simulink model "SecRwLtStCalib"  (R2024b)
settings: Solver=FixedStepDiscrete  StartTime=0.0  StopTime=10.0  FixedStep=0.01  RelTol=1e-3
model workspace (MAT data in the model file):
  KeSMSwAcsMd6SecRwLtStBkReclnUpwdDnwdPos1Max_Val : Simulink.Parameter (value not decoded)
  KeSMSwAcsMd6SecRwLtStBkReclnUpwdDnwdPos1Min_Val : Simulink.Parameter (value not decoded)
  KeSMSwAcsMd6SecRwLtStBkReclnUpwdDnwdPos1_Val : Simulink.Parameter (value not decoded)
  KeSMSwAcsMd6SecRwLtStBkReclnUpwdDnwdPosMax_Val : Simulink.Parameter (value not decoded)
  KeSMSwAcsMd6SecRwLtStBkReclnUpwdDnwdPosMin_Val : Simulink.Parameter (value not decoded)
  KeSMSwAcsMd6SecRwLtStBkReclnUpwdDnwdPos_Val : Simulink.Parameter (value not decoded)
symbols that are objects in the model workspace (value not decoded): KeSMSwAcsMd6SecRwLtStBkReclnUpwdDnwdPos1_Val, KeSMSwAcsMd6SecRwLtStBkReclnUpwdDnwdPos1Max_Val, KeSMSwAcsMd6SecRwLtStBkReclnUpwdDnwdPos1Min_Val, KeSMSwAcsMd6SecRwLtStBkReclnUpwdDnwdPos_Val, KeSMSwAcsMd6SecRwLtStBkReclnUpwdDnwdPosMax_Val, KeSMSwAcsMd6SecRwLtStBkReclnUpwdDnwdPosMin_Val
undefined symbols (not defined in the file or in its folder): KeSMSw4SAcsMd21SecRwLtStBkReclnUpwdDnwdPos_Val, KeSMSw4SAcsMd21SecRwLtStBkReclnUpwdDnwdPosMax_Val, KeSMSw4SAcsMd21SecRwLtStBkReclnUpwdDnwdPosMin_Val, KeSMSw4SAcsMd21SecRwLtStFrwdBkwdPos_Val, KeSMSw4SAcsMd21SecRwLtStFrwdBkwdPosMax_Val, KeSMSw4SAcsMd21SecRwLtStFrwdBkwdPosMin_Val, KeSMSw4SAcsMd21SecRwLtStHdrstFrwdBkwdPos_Val, KeSMSw4SAcsMd21SecRwLtStHdrstFrwdBkwdPosMax_Val, KeSMSw4SAcsMd21SecRwLtStHdrstFrwdBkwdPosMin_Val, KeSMSw4SAcsMd21SecRwLtStHdrstUpwdDnwdPos_Val, KeSMSw4SAcsMd21SecRwLtStHdrstUpwdDnwdPosMax_Val, KeSMSw4SAcsMd21SecRwLtStHdrstUpwdDnwdPosMin_Val, KeSMSw4SAcsMd22SecRwLtStBkReclnUpwdDnwdPos1_Val, KeSMSw4SAcsMd22SecRwLtStBkReclnUpwdDnwdPos2_Val, KeSMSw4SAcsMd22SecRwLtStBkReclnUpwdDnwdPos2Max_Val, KeSMSw4SAcsMd22SecRwLtStBkReclnUpwdDnwdPos2Min_Val, KeSMSw4SAcsMd22SecRwLtStBkReclnUpwdDnwdPosMax_Val, KeSMSw4SAcsMd22SecRwLtStBkReclnUpwdDnwdPosMin_Val, KeSMSw4SAcsMd22SecRwLtStFrwdBkwdPos_Val, KeSMSw4SAcsMd22SecRwLtStFrwdBkwdPosMax_Val, KeSMSw4SAcsMd22SecRwLtStFrwdBkwdPosMin_Val, KeSMSw4SAcsMd22SecRwLtStFtrstUpwdDnwdPos_Val, KeSMSw4SAcsMd22SecRwLtStFtrstUpwdDnwdPosMax_Val, KeSMSw4SAcsMd22SecRwLtStFtrstUpwdDnwdPosMin_Val, KeSMSw4SAcsMd22SecRwLtStHdrstFrwdBkwdPos_Val, KeSMSw4SAcsMd22SecRwLtStHdrstFrwdBkwdPosMax_Val, KeSMSw4SAcsMd22SecRwLtStHdrstFrwdBkwdPosMin_Val, KeSMSw4SAcsMd22SecRwLtStHdrstUpwdDnwdPos_Val, KeSMSw4SAcsMd22SecRwLtStHdrstUpwdDnwdPosMax_Val, KeSMSw4SAcsMd22SecRwLtStHdrstUpwdDnwdPosMin_Val, KeSMSw4SAcsMd22SecRwLtStLegrstOtwdInwdPos_Val, KeSMSw4SAcsMd22SecRwLtStLegrstOtwdInwdPosMax_Val, KeSMSw4SAcsMd22SecRwLtStLegrstOtwdInwdPosMin_Val, KeSMSw4SAcsMd22SecRwLtStLegrstUpwdDnwdPos_Val, KeSMSw4SAcsMd22SecRwLtStLegrstUpwdDnwdPosMax_Val, KeSMSw4SAcsMd22SecRwLtStLegrstUpwdDnwdPosMin_Val, KeSMSw4SAcsMd25SecRwLtStBkReclnUpwdDnwdPos_Val, KeSMSw4SAcsMd25SecRwLtStBkReclnUpwdDnwdPosMax_Val, KeSMSw4SAcsMd25SecRwLtStBkReclnUpwdDnwdPosMin_Val, KeSMSw4SAcsMd25SecRwLtStFrwdBkwdPos_Val, KeSMSw4SAcsMd25SecRwLtStFrwdBkwdPosMax_Val, KeSMSw4SAcsMd25SecRwLtStFrwdBkwdPosMin_Val, KeSMSw4SAcsMd25SecRwLtStHdrstFrwdBkwdPos_Val, KeSMSw4SAcsMd25SecRwLtStHdrstFrwdBkwdPosMax_Val, KeSMSw4SAcsMd25SecRwLtStHdrstFrwdBkwdPosMin_Val, KeSMSw4SAcsMd25SecRwLtStHdrstUpwdDnwdPos_Val, KeSMSw4SAcsMd25SecRwLtStHdrstUpwdDnwdPosMax_Val, KeSMSw4SAcsMd25SecRwLtStHdrstUpwdDnwdPosMin_Val, KeSMSw4SAcsMd26SecRwLtStBkReclnUpwdDnwdPos_Val, KeSMSw4SAcsMd26SecRwLtStBkReclnUpwdDnwdPosMax_Val, KeSMSw4SAcsMd26SecRwLtStBkReclnUpwdDnwdPosMin_Val, KeSMSw4SAcsMd26SecRwLtStFrwdBkwdPos_Val, KeSMSw4SAcsMd26SecRwLtStFrwdBkwdPosMax_Val, KeSMSw4SAcsMd26SecRwLtStFrwdBkwdPosMin_Val, KeSMSw4SAcsMd26SecRwLtStFtrstUpwdDnwdPos_Val, KeSMSw4SAcsMd26SecRwLtStFtrstUpwdDnwdPosMax_Val, KeSMSw4SAcsMd26SecRwLtStFtrstUpwdDnwdPosMin_Val, KeSMSw4SAcsMd26SecRwLtStHdrstFrwdBkwdPos_Val, KeSMSw4SAcsMd26SecRwLtStHdrstFrwdBkwdPosMax_Val, KeSMSw4SAcsMd26SecRwLtStHdrstFrwdBkwdPosMin_Val ... (+496)
libraries: TrgtPosSelcLib x61, StIsPosChkLib x1, simulink x1
(part 2 of 8)

== system SecRwLtStCalib/SecRwLtStArmScrnTrgtPosSelc_1_Cal_sys ==
  StNumFlg_Is4s_read : Inport
  StNumFlg_Is6s_read : Inport  Port=2
  StNumFlg_Is6s7s_read : Inport  Port=3
  StNumFlg_Is7s_read : Inport  Port=4
  function : TriggerPort  TriggerType=function-call  IsSimulinkFunction=on  FunctionName=SecRwLtStArmScrnTrgtPosSelc_1_Cal  VariantControl=(inherit)
  Ground_1 : Ground
  Ground_2 : Ground
  Terminator_{1..4} (4 alike) : Terminator
  EZER2LArmScrnTrgtPosCalib_TrgtPosArray_write : Outport  VectorParamsAs1DForOutWhenUnconnected=off
      settings: EnsureOutportIsVirtual=on
  EZQR2LArmScrnTrgtPosCalib_TrgtPosArray_write : Outport  Port=2  VectorParamsAs1DForOutWhenUnconnected=off
      settings: EnsureOutportIsVirtual=on
  wires:
  StNumFlg_Is4s_read/1 -> Terminator_1/1
  StNumFlg_Is6s_read/1 -> Terminator_2/1
  StNumFlg_Is6s7s_read/1 -> Terminator_3/1
  StNumFlg_Is7s_read/1 -> Terminator_4/1
  Ground_1/1 -> EZER2LArmScrnTrgtPosCalib_TrgtPosArray_write/1
  Ground_2/1 -> EZQR2LArmScrnTrgtPosCalib_TrgtPosArray_write/1

== system SecRwLtStCalib/SecRwLtStBkReclnTrgtPosSelc_1_Cal_sys ==
  IfVeSMSbSecRwLtStCshnFrntUpwdDnwdMovConfig_Val_read : Inport
  IfVeSMSuThdRwLtStCshnFldUpwdDnwdPos_Val_read : Inport  Port=2
  modestate32_Val_read : Inport  Port=3
  R2LBkReclinFirstStepPassFlg_Val_read : Inport  Port=4
  R2LMdSeatOccupied_Val_read : Inport  Port=5
  StNumFlg_Is4s_read : Inport  Port=6
  StNumFlg_Is6s_read : Inport  Port=7
  StNumFlg_Is6s7s_read : Inport  Port=8
  StNumFlg_Is7s_read : Inport  Port=9
  ThdRwLtStCshnFldStgDone_Val_read : Inport  Port=10
  Md27Target1_Val_read : Inport  Port=11
  Md27Target2_Val_read : Inport  Port=12
  function : TriggerPort  TriggerType=function-call  IsSimulinkFunction=on  FunctionName=SecRwLtStBkReclnTrgtPosSelc_1_Cal  VariantControl=(inherit)
  Subsystem1 : Subsystem
  EZER2LBkReclnUpwdDnwdTrgtPosCalib_TrgtPosArray_write : Outport  VectorParamsAs1DForOutWhenUnconnected=off
  EZER2LBkReclnUpwdDnwdTrgtPosCalib1_TrgtPosArray_write : Outport  Port=2  VectorParamsAs1DForOutWhenUnconnected=off
  EZQR2LBkReclnUpwdDnwdTrgtPosCalib_TrgtPosArray_write : Outport  Port=3  VectorParamsAs1DForOutWhenUnconnected=off
  KeSMSw4SAcsMd21BkReclnUpwdDnwdTrgtPosCalib_TrgtPosArray_write : Outport  Port=4  VectorParamsAs1DForOutWhenUnconnected=off
  KeSMSw4SAcsMd22BkReclnUpwdDnwdTrgtPosCalib_TrgtPosArray_write : Outport  Port=5  VectorParamsAs1DForOutWhenUnconnected=off
  KeSMSw4SAcsMd25BkReclnUpwdDnwdTrgtPosCalib_TrgtPosArray_write : Outport  Port=6  VectorParamsAs1DForOutWhenUnconnected=off
  KeSMSw4SAcsMd26BkReclnUpwdDnwdTrgtPosCalib_TrgtPosArray_write : Outport  Port=7  VectorParamsAs1DForOutWhenUnconnected=off
  KeSMSwMd32R2LBkReclnUpwdDnwdTrgtPosCalib_TrgtPosArray_write : Outport  Port=8  VectorParamsAs1DForOutWhenUnconnected=off
  LyLR2LBkReclnUpwdDnwdTrgtPosCalib_TrgtPosArray_write : Outport  Port=9  VectorParamsAs1DForOutWhenUnconnected=off
  Md56R2LBkReclnUpwdDnwdTrgtPosCalib_TrgtPosArray_write : Outport  Port=10  VectorParamsAs1DForOutWhenUnconnected=off
  Md56R2LBkReclnUpwdDnwdTrgtPosCalib1_TrgtPosArray_write : Outport  Port=11  VectorParamsAs1DForOutWhenUnconnected=off
  Md8R2LBkReclnUpwdDnwdTrgtPosCalib_TrgtPosArray_write : Outport  Port=12  VectorParamsAs1DForOutWhenUnconnected=off
  RecvLR2LBkReclnUpwdDnwdTrgtPosCalib_TrgtPosArray_write : Outport  Port=13  VectorParamsAs1DForOutWhenUnconnected=off
  SecRwLtStBkReclnEnTrigBitMask_Val_write : Outport  Port=14  VectorParamsAs1DForOutWhenUnconnected=off
  VIPLExitR2LBkReclnUpwdDnwdTrgtPosCalib_TrgtPosArray_write : Outport  Port=15  VectorParamsAs1DForOutWhenUnconnected=off
  VIPLR2LBkReclnUpwdDnwdTrgtPosCalib_TrgtPosArray_write : Outport  Port=16  VectorParamsAs1DForOutWhenUnconnected=off
  Md27SecRwLtStBkReclnTrgtPosCalib_TrgtPosArray_write : Outport  Port=17  VectorParamsAs1DForOutWhenUnconnected=off
      settings: EnsureOutportIsVirtual=on
  wires:
  Subsystem1/16(SecRwLtStBkReclnEnTrigBitMask_Val_write) -> SecRwLtStBkReclnEnTrigBitMask_Val_write/1
  Subsystem1/1(EZER2LBkReclnUpwdDnwdTrgtPosCalib_TrgtPosArray_write) -> EZER2LBkReclnUpwdDnwdTrgtPosCalib_TrgtPosArray_write/1
  Subsystem1/2(EZQR2LBkReclnUpwdDnwdTrgtPosCalib_TrgtPosArray_write) -> EZQR2LBkReclnUpwdDnwdTrgtPosCalib_TrgtPosArray_write/1
  Subsystem1/3(KeSMSw4SAcsMd21BkReclnUpwdDnwdTrgtPosCalib_TrgtPosArray_write) -> KeSMSw4SAcsMd21BkReclnUpwdDnwdTrgtPosCalib_TrgtPosArray_write/1
  Subsystem1/4(KeSMSw4SAcsMd22BkReclnUpwdDnwdTrgtPosCalib_TrgtPosArray_write) -> KeSMSw4SAcsMd22BkReclnUpwdDnwdTrgtPosCalib_TrgtPosArray_write/1
  Subsystem1/5(KeSMSw4SAcsMd25BkReclnUpwdDnwdTrgtPosCalib_TrgtPosArray_write) -> KeSMSw4SAcsMd25BkReclnUpwdDnwdTrgtPosCalib_TrgtPosArray_write/1
  Subsystem1/6(KeSMSw4SAcsMd26BkReclnUpwdDnwdTrgtPosCalib_TrgtPosArray_write) -> KeSMSw4SAcsMd26BkReclnUpwdDnwdTrgtPosCalib_TrgtPosArray_write/1
  Subsystem1/7(LyLR2LBkReclnUpwdDnwdTrgtPosCalib_TrgtPosArray_write) -> LyLR2LBkReclnUpwdDnwdTrgtPosCalib_TrgtPosArray_write/1
  Subsystem1/8(RecvLR2LBkReclnUpwdDnwdTrgtPosCalib_TrgtPosArray_write) -> RecvLR2LBkReclnUpwdDnwdTrgtPosCalib_TrgtPosArray_write/1
  Subsystem1/9(VIPLR2LBkReclnUpwdDnwdTrgtPosCalib_TrgtPosArray_write) -> VIPLR2LBkReclnUpwdDnwdTrgtPosCalib_TrgtPosArray_write/1
  Subsystem1/10(EZER2LBkReclnUpwdDnwdTrgtPosCalib1_TrgtPosArray_write) -> EZER2LBkReclnUpwdDnwdTrgtPosCalib1_TrgtPosArray_write/1
  Subsystem1/11(VIPLExitR2LBkReclnUpwdDnwdTrgtPosCalib_TrgtPosArray_write) -> VIPLExitR2LBkReclnUpwdDnwdTrgtPosCalib_TrgtPosArray_write/1
  Subsystem1/12(KeSMSwMd32R2LBkReclnUpwdDnwdTrgtPosCalib_TrgtPosArray_write) -> KeSMSwMd32R2LBkReclnUpwdDnwdTrgtPosCalib_TrgtPosArray_write/1
  Subsystem1/13(Md8R2LBkReclnUpwdDnwdTrgtPosCalib_TrgtPosArray_write) -> Md8R2LBkReclnUpwdDnwdTrgtPosCalib_TrgtPosArray_write/1
  Subsystem1/15(Md56R2LBkReclnUpwdDnwdTrgtPosCalib1_TrgtPosArray_write) -> Md56R2LBkReclnUpwdDnwdTrgtPosCalib1_TrgtPosArray_write/1
  Subsystem1/14(Md56R2LBkReclnUpwdDnwdTrgtPosCalib_TrgtPosArray_write) -> Md56R2LBkReclnUpwdDnwdTrgtPosCalib_TrgtPosArray_write/1
  IfVeSMSbSecRwLtStCshnFrntUpwdDnwdMovConfig_Val_read/1 -> Subsystem1/8(IfVeSMSbSecRwLtStCshnFrntUpwdDnwdMovConfig_Val_read)
  IfVeSMSuThdRwLtStCshnFldUpwdDnwdPos_Val_read/1 -> Subsystem1/10(IfVeSMSuThdRwLtStCshnFldUpwdDnwdPos_Val_read)
  ThdRwLtStCshnFldStgDone_Val_read/1 -> Subsystem1/9(ThdRwLtStCshnFldStgDone_Val_read)
  R2LBkReclinFirstStepPassFlg_Val_read/1 -> Subsystem1/7(R2LBkReclinFirstStepPassFlg_Val_read)
  modestate32_Val_read/1 -> Subsystem1/6(modestate32_Val_read)
  R2LMdSeatOccupied_Val_read/1 -> Subsystem1/5(R2LMdSeatOccupied_Val_read)
  StNumFlg_Is4s_read/1 -> Subsystem1/1(StNumFlg_Is4s_read)
  StNumFlg_Is7s_read/1 -> Subsystem1/4(StNumFlg_Is7s_read)
  StNumFlg_Is6s7s_read/1 -> Subsystem1/3(StNumFlg_Is6s7s_read)
  StNumFlg_Is6s_read/1 -> Subsystem1/2(StNumFlg_Is6s_read)
  Md27Target1_Val_read/1 -> Subsystem1/11(Md27Target1_Val_read)
  Md27Target2_Val_read/1 -> Subsystem1/12(Md27Target2_Val_read)
  Subsystem1/17(Md27SecRwLtStBkReclnTrgtPosCalib_TrgtPosArray_write) -> Md27SecRwLtStBkReclnTrgtPosCalib_TrgtPosArray_write/1

== system SecRwLtStCalib/SecRwLtStCalib_Init ==
  Event Listener : EventListener  EventName=reset

== system SecRwLtStCalib/SecRwLtStFtrstTrgtPosSelc_1_Cal_sys ==
  StNumFlg_Is4s_read : Inport
  StNumFlg_Is6s_read : Inport  Port=2
  StNumFlg_Is6s7s_read : Inport  Port=3
  StNumFlg_Is7s_read : Inport  Port=4
  function : TriggerPort  TriggerType=function-call  IsSimulinkFunction=on  FunctionName=SecRwLtStFtrstTrgtPosSelc_1_Cal  VariantControl=(inherit)
  Ground_{1..7} (7 alike) : Ground
  Terminator_{1..4} (4 alike) : Terminator
  KeSMSw4SAcsMd22FtrstTrgtPosCalib_TrgtPosArray_write : Outport  VectorParamsAs1DForOutWhenUnconnected=off
      settings: EnsureOutportIsVirtual=on
  KeSMSw4SAcsMd26FtrstTrgtPosCalib_TrgtPosArray_write : Outport  Port=2  VectorParamsAs1DForOutWhenUnconnected=off
      settings: EnsureOutportIsVirtual=on
  LgrstCloseLR2LFtrstTrgtPosCalib_TrgtPosArray_write : Outport  Port=3  VectorParamsAs1DForOutWhenUnconnected=off
      settings: EnsureOutportIsVirtual=on
  LgrstOpenLR2LFtrstTrgtPosCalib_TrgtPosArray_write : Outport  Port=4  VectorParamsAs1DForOutWhenUnconnected=off
      settings: EnsureOutportIsVirtual=on
  LyLR2LFtrstTrgtPosCalib_TrgtPosArray_write : Outport  Port=5  VectorParamsAs1DForOutWhenUnconnected=off
      settings: EnsureOutportIsVirtual=on
  RecvLR2LFtrstTrgtPosCalib_TrgtPosArray_write : Outport  Port=6  VectorParamsAs1DForOutWhenUnconnected=off
      settings: EnsureOutportIsVirtual=on
  VIPLR2LFtrstTrgtPosCalib_TrgtPosArray_write : Outport  Port=7  VectorParamsAs1DForOutWhenUnconnected=off
      settings: EnsureOutportIsVirtual=on
  wires:
  StNumFlg_Is4s_read/1 -> Terminator_1/1
  StNumFlg_Is6s_read/1 -> Terminator_2/1
  StNumFlg_Is6s7s_read/1 -> Terminator_3/1
  StNumFlg_Is7s_read/1 -> Terminator_4/1
  Ground_1/1 -> KeSMSw4SAcsMd22FtrstTrgtPosCalib_TrgtPosArray_write/1
  Ground_2/1 -> KeSMSw4SAcsMd26FtrstTrgtPosCalib_TrgtPosArray_write/1
  Ground_3/1 -> LgrstCloseLR2LFtrstTrgtPosCalib_TrgtPosArray_write/1
  Ground_4/1 -> LgrstOpenLR2LFtrstTrgtPosCalib_TrgtPosArray_write/1
  Ground_5/1 -> LyLR2LFtrstTrgtPosCalib_TrgtPosArray_write/1
  Ground_6/1 -> RecvLR2LFtrstTrgtPosCalib_TrgtPosArray_write/1
  Ground_7/1 -> VIPLR2LFtrstTrgtPosCalib_TrgtPosArray_write/1

== system SecRwLtStCalib/SecRwLtStFwdBkwdTrgtPosSelc_1_Cal_sys ==
  note: Added blocks
  note: Added blocks
  note: Added blocks
  IfVeSMSbSecRwLtStCshnFrntUpwdDnwdMovConfig_Val_read : Inport
  IfVeSMSuSecRwRtStFrwdBkwdPos_Val_read : Inport  Port=2
  IfVeSMSuSecRwRtStFrwdBkwdPosV_Val_read : Inport  Port=3
  StNumFlg_Is4s_read : Inport  Port=4
  StNumFlg_Is6s_read : Inport  Port=5
  StNumFlg_Is6s7s_read : Inport  Port=6
  StNumFlg_Is7s_read : Inport  Port=7
  function : TriggerPort  TriggerType=function-call  IsSimulinkFunction=on  FunctionName=SecRwLtStFwdBkwdTrgtPosSelc_1_Cal  VariantControl=(inherit)
  PA_KeSMSwAcsMd6SecRwLtStBkReclnUpwdDnwdPos1Max_Val : Constant  Value=KeSMSwAcsMd6SecRwLtStBkReclnUpwdDnwdPos1Max_Val
  PA_KeSMSwAcsMd6SecRwLtStBkReclnUpwdDnwdPos1Min_Val : Constant  Value=KeSMSwAcsMd6SecRwLtStBkReclnUpwdDnwdPos1Min_Val
  PA_KeSMSwAcsMd6SecRwLtStBkReclnUpwdDnwdPos1_Val : Constant  Value=KeSMSwAcsMd6SecRwLtStBkReclnUpwdDnwdPos1_Val
  PA_KeSMSwAcsMd6SecRwLtStBkReclnUpwdDnwdPosMax_Val : Constant  Value=KeSMSwAcsMd6SecRwLtStBkReclnUpwdDnwdPosMax_Val
  PA_KeSMSwAcsMd6SecRwLtStBkReclnUpwdDnwdPosMin_Val : Constant  Value=KeSMSwAcsMd6SecRwLtStBkReclnUpwdDnwdPosMin_Val
  Subsystem2 : Subsystem
  Terminator_{495..499} (5 alike) : Terminator
  EZER2LFwdBkwdTrgtPosCalib_TrgtPosArray_write : Outport  VectorParamsAs1DForOutWhenUnconnected=off
  EZQR2LFwdBkwdTrgtPosCalib_TrgtPosArray_write : Outport  Port=2  VectorParamsAs1DForOutWhenUnconnected=off
  FamlyLR2LFwdBkwdTrgtPosCalib_TrgtPosArray_write : Outport  Port=3  VectorParamsAs1DForOutWhenUnconnected=off
  FamlyRR2LFwdBkwdTrgtPosCalib_TrgtPosArray_write : Outport  Port=4  VectorParamsAs1DForOutWhenUnconnected=off
  INTMLR2LFwdBkwdTrgtPosCalib_TrgtPosArray_write : Outport  Port=5  VectorParamsAs1DForOutWhenUnconnected=off
  KeSMSw4SAcsMd21FwdBkwdTrgtPosCalib_TrgtPosArray_write : Outport  Port=6  VectorParamsAs1DForOutWhenUnconnected=off
  KeSMSw4SAcsMd22FwdBkwdTrgtPosCalib_TrgtPosArray_write : Outport  Port=7  VectorParamsAs1DForOutWhenUnconnected=off
  KeSMSw4SAcsMd25FwdBkwdTrgtPosCalib_TrgtPosArray_write : Outport  Port=8  VectorParamsAs1DForOutWhenUnconnected=off
  KeSMSw4SAcsMd26FwdBkwdTrgtPosCalib_TrgtPosArray_write : Outport  Port=9  VectorParamsAs1DForOutWhenUnconnected=off
  KeSMSw4sLegrstOpenLMdFwdBkwdTrgtPosCalib_TrgtPosArray_write : Outport  Port=10  VectorParamsAs1DForOutWhenUnconnected=off
  KeSMSw4SLyingLMDFwdBkwdTrgtPosCalib_TrgtPosArray_write : Outport  Port=11  VectorParamsAs1DForOutWhenUnconnected=off
  KeSMSw4SVIPLMDFwdBkwdTrgtPosCalib_TrgtPosArray_write : Outport  Port=12  VectorParamsAs1DForOutWhenUnconnected=off
  Md56R2LFwdBkwdTrgtPosCalib_TrgtPosArray_write : Outport  Port=13  VectorParamsAs1DForOutWhenUnconnected=off
  Md8R2LFwdBkwdTrgtPosCalib_TrgtPosArray_write : Outport  Port=14  VectorParamsAs1DForOutWhenUnconnected=off
  SecRwLtStFwdBkwdEnTrigBitMask_Val_write : Outport  Port=15  VectorParamsAs1DForOutWhenUnconnected=off
  VIPLExitR2LFwdBkwdTrgtPosCalib_TrgtPosArray_write : Outport  Port=16  VectorParamsAs1DForOutWhenUnconnected=off
  VIPLR2LFwdBkwdTrgtPosCalib_TrgtPosArray_write : Outport  Port=17  VectorParamsAs1DForOutWhenUnconnected=off
  wires:
  Subsystem2/17(SecRwLtStFwdBkwdEnTrigBitMask_Val_write) -> SecRwLtStFwdBkwdEnTrigBitMask_Val_write/1
  Subsystem2/1(EZER2LFwdBkwdTrgtPosCalib_TrgtPosArray_write) -> EZER2LFwdBkwdTrgtPosCalib_TrgtPosArray_write/1
  Subsystem2/2(EZQR2LFwdBkwdTrgtPosCalib_TrgtPosArray_write) -> EZQR2LFwdBkwdTrgtPosCalib_TrgtPosArray_write/1
  Subsystem2/3(FamlyLR2LFwdBkwdTrgtPosCalib_TrgtPosArray_write) -> FamlyLR2LFwdBkwdTrgtPosCalib_TrgtPosArray_write/1
  Subsystem2/4(FamlyRR2LFwdBkwdTrgtPosCalib_TrgtPosArray_write) -> FamlyRR2LFwdBkwdTrgtPosCalib_TrgtPosArray_write/1
  Subsystem2/5(INTMLR2LFwdBkwdTrgtPosCalib_TrgtPosArray_write) -> INTMLR2LFwdBkwdTrgtPosCalib_TrgtPosArray_write/1
  Subsystem2/6(KeSMSw4SAcsMd21FwdBkwdTrgtPosCalib_TrgtPosArray_write) -> KeSMSw4SAcsMd21FwdBkwdTrgtPosCalib_TrgtPosArray_write/1
  Subsystem2/7(KeSMSw4SAcsMd22FwdBkwdTrgtPosCalib_TrgtPosArray_write) -> KeSMSw4SAcsMd22FwdBkwdTrgtPosCalib_TrgtPosArray_write/1
  Subsystem2/8(KeSMSw4SAcsMd25FwdBkwdTrgtPosCalib_TrgtPosArray_write) -> KeSMSw4SAcsMd25FwdBkwdTrgtPosCalib_TrgtPosArray_write/1
  Subsystem2/9(KeSMSw4SAcsMd26FwdBkwdTrgtPosCalib_TrgtPosArray_write) -> KeSMSw4SAcsMd26FwdBkwdTrgtPosCalib_TrgtPosArray_write/1
  Subsystem2/10(VIPLR2LFwdBkwdTrgtPosCalib_TrgtPosArray_write) -> VIPLR2LFwdBkwdTrgtPosCalib_TrgtPosArray_write/1
  Subsystem2/11(KeSMSw4sLegrstOpenLMdFwdBkwdTrgtPosCalib_TrgtPosArray_write) -> KeSMSw4sLegrstOpenLMdFwdBkwdTrgtPosCalib_TrgtPosArray_write/1
  Subsystem2/12(KeSMSw4SLyingLMDFwdBkwdTrgtPosCalib_TrgtPosArray_write) -> KeSMSw4SLyingLMDFwdBkwdTrgtPosCalib_TrgtPosArray_write/1
  Subsystem2/16(Md56R2LFwdBkwdTrgtPosCalib_TrgtPosArray_write) -> Md56R2LFwdBkwdTrgtPosCalib_TrgtPosArray_write/1
  Subsystem2/15(Md8R2LFwdBkwdTrgtPosCalib_TrgtPosArray_write) -> Md8R2LFwdBkwdTrgtPosCalib_TrgtPosArray_write/1
  Subsystem2/14(VIPLExitR2LFwdBkwdTrgtPosCalib_TrgtPosArray_write) -> VIPLExitR2LFwdBkwdTrgtPosCalib_TrgtPosArray_write/1
  Subsystem2/13(KeSMSw4SVIPLMDFwdBkwdTrgtPosCalib_TrgtPosArray_write) -> KeSMSw4SVIPLMDFwdBkwdTrgtPosCalib_TrgtPosArray_write/1
  IfVeSMSuSecRwRtStFrwdBkwdPos_Val_read/1 -> Subsystem2/1(IfVeSMSuSecRwRtStFrwdBkwdPos_Val_read)
  IfVeSMSuSecRwRtStFrwdBkwdPosV_Val_read/1 -> Subsystem2/2(IfVeSMSuSecRwRtStFrwdBkwdPosV_Val_read)
  StNumFlg_Is4s_read/1 -> Subsystem2/3(StNumFlg_Is4s_read)
  StNumFlg_Is6s_read/1 -> Subsystem2/4(StNumFlg_Is6s_read)
  StNumFlg_Is6s7s_read/1 -> Subsystem2/5(StNumFlg_Is6s7s_read)
  StNumFlg_Is7s_read/1 -> Subsystem2/6(StNumFlg_Is7s_read)
  IfVeSMSbSecRwLtStCshnFrntUpwdDnwdMovConfig_Val_read/1 -> Subsystem2/7(IfVeSMSbSecRwLtStCshnFrntUpwdDnwdMovConfig_Val_read)

== system SecRwLtStCalib/SecRwLtStHdrstFwdBkwdTrgtPosSelc_1_Cal_sys ==
  IfVeSMSuHeightIndexLt_Val_read : Inport
  StNumFlg_Is4s_read : Inport  Port=2
  StNumFlg_Is6s_read : Inport  Port=3
  StNumFlg_Is6s7s_read : Inport  Port=4
  StNumFlg_Is7s_read : Inport  Port=5
  function : TriggerPort  TriggerType=function-call  IsSimulinkFunction=on  FunctionName=SecRwLtStHdrstFwdBkwdTrgtPosSelc_1_Cal  VariantControl=(inherit)
  Ground_{1..7} (7 alike) : Ground
  Terminator_{1..5} (5 alike) : Terminator
  KeSMSw4SAcsMd21HdrstFwdBkwdTrgtPosCalib_TrgtPosArray_write : Outport  VectorParamsAs1DForOutWhenUnconnected=off
      settings: EnsureOutportIsVirtual=on
  KeSMSw4SAcsMd22HdrstFwdBkwdTrgtPosCalib_TrgtPosArray_write : Outport  Port=2  VectorParamsAs1DForOutWhenUnconnected=off
      settings: EnsureOutportIsVirtual=on
  KeSMSw4SAcsMd25HdrstFwdBkwdTrgtPosCalib_TrgtPosArray_write : Outport  Port=3  VectorParamsAs1DForOutWhenUnconnected=off
      settings: EnsureOutportIsVirtual=on
  KeSMSw4SAcsMd26HdrstFwdBkwdTrgtPosCalib_TrgtPosArray_write : Outport  Port=4  VectorParamsAs1DForOutWhenUnconnected=off
      settings: EnsureOutportIsVirtual=on
  LyLR2LHdrstFwdBkwdTrgtPosCalib_TrgtPosArray_write : Outport  Port=5  VectorParamsAs1DForOutWhenUnconnected=off
      settings: EnsureOutportIsVirtual=on
  RecvLR2LHdrstFwdBkwdTrgtPosCalib_TrgtPosArray_write : Outport  Port=6  VectorParamsAs1DForOutWhenUnconnected=off
      settings: EnsureOutportIsVirtual=on
  VIPLR2LHdrstFwdBkwdTrgtPosCalib_TrgtPosArray_write : Outport  Port=7  VectorParamsAs1DForOutWhenUnconnected=off
      settings: EnsureOutportIsVirtual=on
  wires:
  IfVeSMSuHeightIndexLt_Val_read/1 -> Terminator_1/1
  StNumFlg_Is4s_read/1 -> Terminator_2/1
  StNumFlg_Is6s_read/1 -> Terminator_3/1
  StNumFlg_Is6s7s_read/1 -> Terminator_4/1
  StNumFlg_Is7s_read/1 -> Terminator_5/1
  Ground_1/1 -> KeSMSw4SAcsMd21HdrstFwdBkwdTrgtPosCalib_TrgtPosArray_write/1
  Ground_2/1 -> KeSMSw4SAcsMd22HdrstFwdBkwdTrgtPosCalib_TrgtPosArray_write/1
  Ground_3/1 -> KeSMSw4SAcsMd25HdrstFwdBkwdTrgtPosCalib_TrgtPosArray_write/1
  Ground_4/1 -> KeSMSw4SAcsMd26HdrstFwdBkwdTrgtPosCalib_TrgtPosArray_write/1
  Ground_5/1 -> LyLR2LHdrstFwdBkwdTrgtPosCalib_TrgtPosArray_write/1
  Ground_6/1 -> RecvLR2LHdrstFwdBkwdTrgtPosCalib_TrgtPosArray_write/1
  Ground_7/1 -> VIPLR2LHdrstFwdBkwdTrgtPosCalib_TrgtPosArray_write/1

== system SecRwLtStCalib/SecRwLtStHdrstUpwdDnwdTrgtPosSelc_1_Cal_sys ==
  IfVeSMSuHeightIndexLt_Val_read : Inport
  StNumFlg_Is4s_read : Inport  Port=2
  StNumFlg_Is6s_read : Inport  Port=3
  StNumFlg_Is6s7s_read : Inport  Port=4
  StNumFlg_Is7s_read : Inport  Port=5
  function : TriggerPort  TriggerType=function-call  IsSimulinkFunction=on  FunctionName=SecRwLtStHdrstUpwdDnwdTrgtPosSelc_1_Cal  VariantControl=(inherit)
  Ground_{1..7} (7 alike) : Ground
  Terminator_{1..5} (5 alike) : Terminator
  KeSMSw4SAcsMd21HdrstUpwdDnwdTrgtPosCalib_TrgtPosArray_write : Outport  VectorParamsAs1DForOutWhenUnconnected=off
      settings: EnsureOutportIsVirtual=on
  KeSMSw4SAcsMd22HdrstUpwdDnwdTrgtPosCalib_TrgtPosArray_write : Outport  Port=2  VectorParamsAs1DForOutWhenUnconnected=off
      settings: EnsureOutportIsVirtual=on
  KeSMSw4SAcsMd25HdrstUpwdDnwdTrgtPosCalib_TrgtPosArray_write : Outport  Port=3  VectorParamsAs1DForOutWhenUnconnected=off
      settings: EnsureOutportIsVirtual=on
  KeSMSw4SAcsMd26HdrstUpwdDnwdTrgtPosCalib_TrgtPosArray_write : Outport  Port=4  VectorParamsAs1DForOutWhenUnconnected=off
      settings: EnsureOutportIsVirtual=on
  LyLR2LHdrstUpwdDnwdTrgtPosCalib_TrgtPosArray_write : Outport  Port=5  VectorParamsAs1DForOutWhenUnconnected=off
      settings: EnsureOutportIsVirtual=on
  RecvLR2LHdrstUpwdDnwdTrgtPosCalib_TrgtPosArray_write : Outport  Port=6  VectorParamsAs1DForOutWhenUnconnected=off
      settings: EnsureOutportIsVirtual=on
  VIPLR2LHdrstUpwdDnwdTrgtPosCalib_TrgtPosArray_write : Outport  Port=7  VectorParamsAs1DForOutWhenUnconnected=off
      settings: EnsureOutportIsVirtual=on
  wires:
  IfVeSMSuHeightIndexLt_Val_read/1 -> Terminator_1/1
  StNumFlg_Is4s_read/1 -> Terminator_2/1
  StNumFlg_Is6s_read/1 -> Terminator_3/1
  StNumFlg_Is6s7s_read/1 -> Terminator_4/1
  StNumFlg_Is7s_read/1 -> Terminator_5/1
  Ground_1/1 -> KeSMSw4SAcsMd21HdrstUpwdDnwdTrgtPosCalib_TrgtPosArray_write/1
  Ground_2/1 -> KeSMSw4SAcsMd22HdrstUpwdDnwdTrgtPosCalib_TrgtPosArray_write/1
  Ground_3/1 -> KeSMSw4SAcsMd25HdrstUpwdDnwdTrgtPosCalib_TrgtPosArray_write/1
  Ground_4/1 -> KeSMSw4SAcsMd26HdrstUpwdDnwdTrgtPosCalib_TrgtPosArray_write/1
  Ground_5/1 -> LyLR2LHdrstUpwdDnwdTrgtPosCalib_TrgtPosArray_write/1
  Ground_6/1 -> RecvLR2LHdrstUpwdDnwdTrgtPosCalib_TrgtPosArray_write/1
  Ground_7/1 -> VIPLR2LHdrstUpwdDnwdTrgtPosCalib_TrgtPosArray_write/1

== system SecRwLtStCalib/SecRwLtStLgrstInwdOtwdTrgtPosSelc_1_Cal_sys ==
  IfVeSMSbSecRwLtStCshnFrntUpwdDnwdMovConfig_Val_read : Inport
  IfVeSMSuHeightIndexLt_Val_read : Inport  Port=2
  StNumFlg_Is4s_read : Inport  Port=3
  StNumFlg_Is6s_read : Inport  Port=4
  StNumFlg_Is6s7s_read : Inport  Port=5
  StNumFlg_Is7s_read : Inport  Port=6
  function : TriggerPort  TriggerType=function-call  IsSimulinkFunction=on  FunctionName=SecRwLtStLgrstInwdOtwdTrgtPosSelc_1_Cal  VariantControl=(inherit)
  Subsystem2 : Subsystem
  KeSMSw4SAcsMd22LgrstInwdOtwdTrgtPosCalib_TrgtPosArray_write : Outport  VectorParamsAs1DForOutWhenUnconnected=off
  KeSMSw4SAcsMd26LgrstInwdOtwdTrgtPosCalib_TrgtPosArray_write : Outport  Port=2  VectorParamsAs1DForOutWhenUnconnected=off
  KeSMSwEZEEntryLgrstInwdOtwdTrgtPosCalib_TrgtPosArray_write : Outport  Port=3  VectorParamsAs1DForOutWhenUnconnected=off
  LgrstCloseLR2LLgrstInwdOtwdTrgtPosCalib_TrgtPosArray_write : Outport  Port=4  VectorParamsAs1DForOutWhenUnconnected=off
  LgrstOpen4sLR2LLgrstInwdOtwdTrgtPosCalib_TrgtPosArray_write : Outport  Port=5  VectorParamsAs1DForOutWhenUnconnected=off
  LyLR2LLgrstInwdOtwdTrgtPosCalib_TrgtPosArray_write : Outport  Port=6  VectorParamsAs1DForOutWhenUnconnected=off
  Md56LgrstInwdOtwdTrgtPosCalib_TrgtPosArray_write : Outport  Port=7  VectorParamsAs1DForOutWhenUnconnected=off
  Md8R2LLgrstInwdOtwdTrgtPosCalib_TrgtPosArray_write : Outport  Port=8  VectorParamsAs1DForOutWhenUnconnected=off
  RecvLR2LLgrstInwdOtwdTrgtPosCalib_TrgtPosArray_write : Outport  Port=9  VectorParamsAs1DForOutWhenUnconnected=off
  SecRwLtStLgrstInwdOtwdEnTrigBitMask_Val_write : Outport  Port=10  VectorParamsAs1DForOutWhenUnconnected=off
  VIP4sLR2LLgrstInwdOtwdTrgtPosCalib_TrgtPosArray_write : Outport  Port=11  VectorParamsAs1DForOutWhenUnconnected=off
  VIPLExitR2LLgrstInwdOtwdTrgtPosCalib_TrgtPosArray_write : Outport  Port=12  VectorParamsAs1DForOutWhenUnconnected=off
  VIPLR2LLgrstInwdOtwdTrgtPosCalib_TrgtPosArray_write : Outport  Port=13  VectorParamsAs1DForOutWhenUnconnected=off
  wires:
  Subsystem2/13(SecRwLtStLgrstInwdOtwdEnTrigBitMask_Val_write) -> SecRwLtStLgrstInwdOtwdEnTrigBitMask_Val_write/1
  Subsystem2/1(LgrstCloseLR2LLgrstInwdOtwdTrgtPosCalib_TrgtPosArray_write) -> LgrstCloseLR2LLgrstInwdOtwdTrgtPosCalib_TrgtPosArray_write/1
  Subsystem2/2(LgrstOpen4sLR2LLgrstInwdOtwdTrgtPosCalib_TrgtPosArray_write) -> LgrstOpen4sLR2LLgrstInwdOtwdTrgtPosCalib_TrgtPosArray_write/1
  Subsystem2/3(LyLR2LLgrstInwdOtwdTrgtPosCalib_TrgtPosArray_write) -> LyLR2LLgrstInwdOtwdTrgtPosCalib_TrgtPosArray_write/1
  Subsystem2/4(RecvLR2LLgrstInwdOtwdTrgtPosCalib_TrgtPosArray_write) -> RecvLR2LLgrstInwdOtwdTrgtPosCalib_TrgtPosArray_write/1
  Subsystem2/5(VIP4sLR2LLgrstInwdOtwdTrgtPosCalib_TrgtPosArray_write) -> VIP4sLR2LLgrstInwdOtwdTrgtPosCalib_TrgtPosArray_write/1
  Subsystem2/6(KeSMSw4SAcsMd22LgrstInwdOtwdTrgtPosCalib_TrgtPosArray_write) -> KeSMSw4SAcsMd22LgrstInwdOtwdTrgtPosCalib_TrgtPosArray_write/1
  Subsystem2/7(KeSMSw4SAcsMd26LgrstInwdOtwdTrgtPosCalib_TrgtPosArray_write) -> KeSMSw4SAcsMd26LgrstInwdOtwdTrgtPosCalib_TrgtPosArray_write/1
  Subsystem2/8(VIPLR2LyLgrstInwdOtwdTrgtPosCalib_TrgtPosArray_write) -> VIPLR2LLgrstInwdOtwdTrgtPosCalib_TrgtPosArray_write/1
  Subsystem2/9(VIPLExitR2LLgrstInwdOtwdTrgtPosCalib_TrgtPosArray_write) -> VIPLExitR2LLgrstInwdOtwdTrgtPosCalib_TrgtPosArray_write/1
  Subsystem2/10(KeSMSwEZEEntryLgrstInwdOtwdTrgtPosCalib_TrgtPosArray_write) -> KeSMSwEZEEntryLgrstInwdOtwdTrgtPosCalib_TrgtPosArray_write/1
  Subsystem2/11(Md8R2LLgrstInwdOtwdTrgtPosCalib_TrgtPosArray_write) -> Md8R2LLgrstInwdOtwdTrgtPosCalib_TrgtPosArray_write/1
  Subsystem2/12(Md56LgrstInwdOtwdTrgtPosCalib_TrgtPosArray_write) -> Md56LgrstInwdOtwdTrgtPosCalib_TrgtPosArray_write/1
  IfVeSMSbSecRwLtStCshnFrntUpwdDnwdMovConfig_Val_read/1 -> Subsystem2/6(IfVeSMSbSecRwLtStCshnFrntUpwdDnwdMovConfig_Val_read)
  IfVeSMSuHeightIndexLt_Val_read/1 -> Subsystem2/1(IfVeSMSuHeightIndexLt_Val_read)
  StNumFlg_Is4s_read/1 -> Subsystem2/2(StNumFlg_Is4s_read)
  StNumFlg_Is6s_read/1 -> Subsystem2/3(StNumFlg_Is6s_read)
  StNumFlg_Is6s7s_read/1 -> Subsystem2/4(StNumFlg_Is6s7s_read)
  StNumFlg_Is7s_read/1 -> Subsystem2/5(StNumFlg_Is7s_read)

== system SecRwLtStCalib/SecRwLtStLgrstUpwdDnwdTrgtPosSelc_1_Cal_sys ==
  IfVeSMSbSecRwLtStCshnFrntUpwdDnwdMovConfig_Val_read : Inport
  StNumFlg_Is4s_read : Inport  Port=2
  StNumFlg_Is6s_read : Inport  Port=3
  StNumFlg_Is6s7s_read : Inport  Port=4
  StNumFlg_Is7s_read : Inport  Port=5
  function : TriggerPort  TriggerType=function-call  IsSimulinkFunction=on  FunctionName=SecRwLtStLgrstUpwdDnwdTrgtPosSelc_1_Cal  VariantControl=(inherit)
  Subsystem1 : Subsystem
  EZER2LLgrstUpwdDnwdTrgtPosCalib_TrgtPosArray_write : Outport  VectorParamsAs1DForOutWhenUnconnected=off
  EZQR2LLgrstUpwdDnwdTrgtPosCalib_TrgtPosArray_write : Outport  Port=2  VectorParamsAs1DForOutWhenUnconnected=off
  KeSMSw4SAcsMd22LgrstUpwdDnwdTrgtPosCalib_TrgtPosArray_write : Outport  Port=3  VectorParamsAs1DForOutWhenUnconnected=off
  KeSMSw4SAcsMd26LgrstUpwdDnwdTrgtPosCalib_TrgtPosArray_write : Outport  Port=4  VectorParamsAs1DForOutWhenUnconnected=off
  LgrstCloseLR2LLgrstUpwdDnwdTrgtPosCalib_TrgtPosArray_write : Outport  Port=5  VectorParamsAs1DForOutWhenUnconnected=off
  LgrstOpenLR2LLgrstUpwdDnwdTrgtPosCalib_TrgtPosArray_write : Outport  Port=6  VectorParamsAs1DForOutWhenUnconnected=off
  LyLR2LLgrstUpwdDnwdTrgtPosCalib_TrgtPosArray_write : Outport  Port=7  VectorParamsAs1DForOutWhenUnconnected=off
  Md56R2LLgrstUpwdDnwdTrgtPosCalib_TrgtPosArray_write : Outport  Port=8  VectorParamsAs1DForOutWhenUnconnected=off
  Md8R2LLgrstUpwdDnwdTrgtPosCalib_TrgtPosArray_write : Outport  Port=9  VectorParamsAs1DForOutWhenUnconnected=off
  RecvLR2LLgrstUpwdDnwdTrgtPosCalib_TrgtPosArray_write : Outport  Port=10  VectorParamsAs1DForOutWhenUnconnected=off
  SecRwLtStLgrstUpwdDnwdEnTrigBitMask_Val_write : Outport  Port=11  VectorParamsAs1DForOutWhenUnconnected=off
  VIPExitLR2LLgrstUpwdDnwdTrgtPosCalib_TrgtPosArray_write : Outport  Port=12  VectorParamsAs1DForOutWhenUnconnected=off
  VIPLR2LLgrstUpwdDnwdTrgtPosCalib_TrgtPosArray_write : Outport  Port=13  VectorParamsAs1DForOutWhenUnconnected=off
      settings: EnsureOutportIsVirtual=on
  wires:
  Subsystem1/13(SecRwLtStLgrstUpwdDnwdEnTrigBitMask_Val_write) -> SecRwLtStLgrstUpwdDnwdEnTrigBitMask_Val_write/1
  Subsystem1/1(EZER2LLgrstUpwdDnwdTrgtPosCalib_TrgtPosArray_write) -> EZER2LLgrstUpwdDnwdTrgtPosCalib_TrgtPosArray_write/1
  Subsystem1/2(EZQR2LLgrstUpwdDnwdTrgtPosCalib_TrgtPosArray_write) -> EZQR2LLgrstUpwdDnwdTrgtPosCalib_TrgtPosArray_write/1
  Subsystem1/3(LgrstCloseLR2LLgrstUpwdDnwdTrgtPosCalib_TrgtPosArray_write) -> LgrstCloseLR2LLgrstUpwdDnwdTrgtPosCalib_TrgtPosArray_write/1
  Subsystem1/4(LgrstOpenLR2LLgrstUpwdDnwdTrgtPosCalib_TrgtPosArray_write) -> LgrstOpenLR2LLgrstUpwdDnwdTrgtPosCalib_TrgtPosArray_write/1
  Subsystem1/5(LyLR2LLgrstUpwdDnwdTrgtPosCalib_TrgtPosArray_write) -> LyLR2LLgrstUpwdDnwdTrgtPosCalib_TrgtPosArray_write/1
  Subsystem1/6(RecvLR2LLgrstUpwdDnwdTrgtPosCalib_TrgtPosArray_write) -> RecvLR2LLgrstUpwdDnwdTrgtPosCalib_TrgtPosArray_write/1
  Subsystem1/7(VIPLR2LLgrstUpwdDnwdTrgtPosCalib_TrgtPosArray_write) -> VIPLR2LLgrstUpwdDnwdTrgtPosCalib_TrgtPosArray_write/1
  Subsystem1/8(KeSMSw4SAcsMd22LgrstUpwdDnwdTrgtPosCalib_TrgtPosArray_write) -> KeSMSw4SAcsMd22LgrstUpwdDnwdTrgtPosCalib_TrgtPosArray_write/1
  Subsystem1/9(KeSMSw4SAcsMd26LgrstUpwdDnwdTrgtPosCalib_TrgtPosArray_write) -> KeSMSw4SAcsMd26LgrstUpwdDnwdTrgtPosCalib_TrgtPosArray_write/1
  Subsystem1/10(VIPExitLR2LLgrstUpwdDnwdTrgtPosCalib_TrgtPosArray_write) -> VIPExitLR2LLgrstUpwdDnwdTrgtPosCalib_TrgtPosArray_write/1
  Subsystem1/11(Md8R2LLgrstUpwdDnwdTrgtPosCalib_TrgtPosArray_write) -> Md8R2LLgrstUpwdDnwdTrgtPosCalib_TrgtPosArray_write/1
  Subsystem1/12(Md56R2LLgrstUpwdDnwdTrgtPosCalib_TrgtPosArray_write) -> Md56R2LLgrstUpwdDnwdTrgtPosCalib_TrgtPosArray_write/1
  IfVeSMSbSecRwLtStCshnFrntUpwdDnwdMovConfig_Val_read/1 -> Subsystem1/5(IfVeSMSbSecRwLtStCshnFrntUpwdDnwdMovConfig_Val_read)
  StNumFlg_Is4s_read/1 -> Subsystem1/1(StNumFlg_Is4s_read)
  StNumFlg_Is6s_read/1 -> Subsystem1/2(StNumFlg_Is6s_read)
  StNumFlg_Is6s7s_read/1 -> Subsystem1/3(StNumFlg_Is6s7s_read)
  StNumFlg_Is7s_read/1 -> Subsystem1/4(StNumFlg_Is7s_read)
